simulink model "Cascade_Realization"  (R2020b)
settings: Solver=FixedStepAuto  StartTime=0.0  StopTime=10.0  FixedStep=1  RelTol=1e-3
PreLoadFcn:
  | vars
values from neighbouring files (symbols this model uses):
  b11 = 1    [vars.m]
  b12 = 2    [vars.m]
  b13 = 1    [vars.m]
  b21 = 1    [vars.m]
  b22 = 1    [vars.m]
  b23 = 1    [vars.m]
settings Model: Creator=hp  LastModifiedBy=hp
settings DataIOCC: SaveOutput=off  SaveTime=off

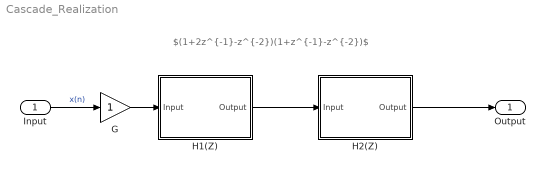
== system Cascade_Realization ==
  note: $(1+2z^{-1}-z^{-2})(1+z^{-1}-z^{-2})$
  Input : Inport  OutDataTypeStr=double  PortDimensions=1  SampleTime=[1,0]
  G : Gain
  H1(Z) : Subsystem
  H2(Z) : Subsystem
  Output : Outport  OutDataTypeStr=double  PortDimensions=1  SampleTime=[1,0]
  wires:
  H1(Z)/1(Output) -> H2(Z)/1(Input)
  H2(Z)/1(Output) -> Output/1
  Input/1 -> G/1  "x(n)"
  G/1 -> H1(Z)/1(Input)

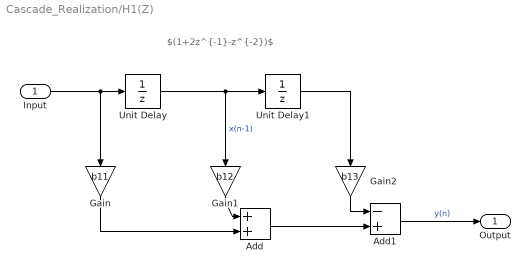
== system Cascade_Realization/H1(Z) ==
  note: $(1+2z^{-1}-z^{-2})$
  Input : Inport
  Add : Sum
  Add1 : Sum  Inputs=-+
  Gain : Gain  Gain=b11
  Gain1 : Gain  Gain=b12
  Gain2 : Gain  Gain=b13
  Unit Delay : UnitDelay  SampleTime=-1  HasFrameUpgradeWarning=on
  Unit Delay1 : UnitDelay  SampleTime=-1  HasFrameUpgradeWarning=on
  Output : Outport
  wires:
  Add1/1 -> Output/1  "y(n)"
  Gain2/1 -> Add1/1
  Input/1 -> Unit Delay/1, Gain/1
  Unit Delay/1 -> Unit Delay1/1, Gain1/1  "x(n-1)"
  Gain/1 -> Add/2
  Add/1 -> Add1/2
  Gain1/1 -> Add/1
  Unit Delay1/1 -> Gain2/1

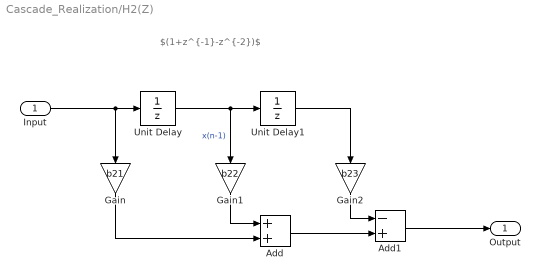
== system Cascade_Realization/H2(Z) ==
  note: $(1+z^{-1}-z^{-2})$
  Input : Inport
  Add : Sum
  Add1 : Sum  Inputs=-+
  Gain : Gain  Gain=b21
  Gain1 : Gain  Gain=b22
  Gain2 : Gain  Gain=b23
  Unit Delay : UnitDelay  SampleTime=-1  HasFrameUpgradeWarning=on
  Unit Delay1 : UnitDelay  SampleTime=-1  HasFrameUpgradeWarning=on
  Output : Outport
  wires:
  Gain1/1 -> Add/1
  Gain2/1 -> Add1/1
  Add/1 -> Add1/2
  Unit Delay1/1 -> Gain2/1
  Gain/1 -> Add/2
  Add1/1 -> Output/1
  Input/1 -> Unit Delay/1, Gain/1
  Unit Delay/1 -> Unit Delay1/1, Gain1/1  "x(n-1)"
